simulink library "DC_Loads_Lib"  (R2021b)
settings: Solver=VariableStepAuto  StartTime=0.0  StopTime=10.0  RelTol=1e-3
undefined symbols (not defined in the file): APN_Param, D1, Delta, Hydride, Metal, Nickel, Ts
libraries: fl_lib x27, nesl_utility x14, spsSeriesRLCBranchLib x8, spsIdealSwitchLib x4, spsCurrentMeasurementLib x4, spsGroundLib x4, spsUniversalBridgeLib x4, spsThreePhaseTransformerThreeWindingsLib x2, spsBatteryLib x1, simulink x1, spsDCMachineLib x1, spsVoltageMeasurementLib x1
Description:
  | Copyright 2019-2021 The MathWorks, Inc.
settings Model: Creator=smiller  LastModifiedBy=janvan
settings SolverCC: AlgebraicLoopSolver=TrustRegion
settings DebuggingCC: SFMachineParentedDataDiag=warning
settings SFSimCC: CustomCodeUndefinedFunction=UseInterfaceOnly

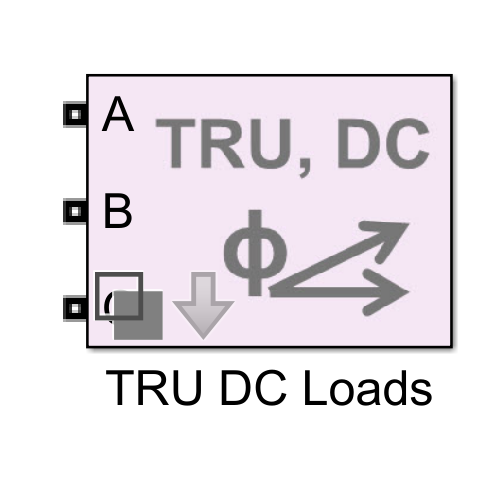
[thumbnail: Simulink's stored preview of the top-level diagram]
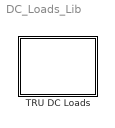
== system DC_Loads_Lib ==
  TRU DC Loads : Subsystem  RequirementInfo={} %GIDa_9ca9392e_c8fd_4c90_afb4_e22deb55bae6  Variant=on  VariantControlMode=label  LabelModeActiveChoice=Phasor  mask{ModelType=Phasor, PQ_Model=Initial}
      mask prompts: ModelType "Model Type"; PQ_Model "PQ Model"
      mask init:
      | set_param(gcb,'LabelModeActiveChoice',get_param(gcb,'ModelType'));
      | set_param([gcb '/Phasor'],'PQ_Model',get_param(gcb,'PQ_Model'));
      settings: AttributesFormatString=%<BlockChoice>
      mask TypeOptions ModelType: Detailed | Multidomain | Phasor
      mask TypeOptions PQ_Model: Initial | Tuned
      mask Display:
      | blk=find_system(gcbh, 'SearchDepth', 1, 'FollowLinks','on','LookUnderMasks','all', 'Parent', gcb,'VariantObject', get_param(gcb,'activevariant'));
      | eval(get_param(blk, 'MaskDisplay'));

== system DC_Loads_Lib/TRU DC Loads ==
  Detailed : Subsystem  VariantControl=Detailed
      mask Display: image('TRU_Detailed_IMAGE.jpg');
  Multidomain : Subsystem  VariantControl=Multidomain
      mask Display: image('TRU_Multidomain_IMAGE.jpg');
  Phasor : Subsystem  VariantControl=Phasor  mask{PQ_Model=Initial}
      mask prompts: PQ_Model "PQ Model"
      mask init:
      | set_param([gcb '/Calc PQ'],'PQ_Model',get_param(gcb,'PQ_Model'));
      mask TypeOptions PQ_Model: Initial | Tuned
      mask Display: image('TRU_Phasor_IMAGE.jpg');
  A : PMIOPort  Side=Left
  B : PMIOPort  Port=2  Side=Left
  C : PMIOPort  Port=3  Side=Left

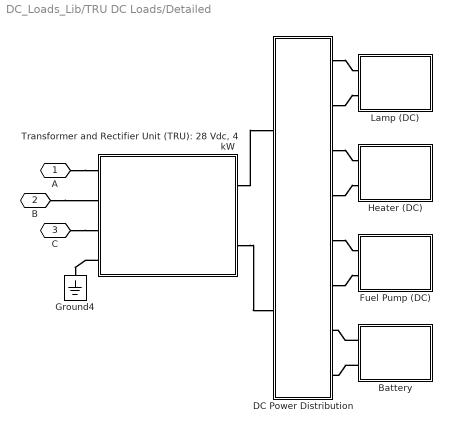
== system DC_Loads_Lib/TRU DC Loads/Detailed ==
  Battery : Subsystem
      mask Display:
      | image(imread('BatteryDC_PS_IMAGE.jpg','jpg'))
      | port_label('LConn',1,'+');
      | port_label('LConn',2,'-');
  "DC Power Distribution " : Subsystem
  Fuel Pump (DC) : Subsystem
      mask Display:
      | image(imread('PumpDC_PS_IMAGE.jpg','jpg'))
      | port_label('LConn',1,'+');
      | port_label('LConn',2,'-');
  Ground4 : spsGroundLib/Ground  LConnTagsString=a
  Heater (DC) : Subsystem
      mask Display:
      | image(imread('HeaterDC_PS_IMAGE.jpg','jpg'))
      | port_label('LConn',1,'+');
      | port_label('LConn',2,'-');
  Lamp (DC) : Subsystem
      mask Display:
      | image(imread('LampDC_PS_IMAGE.jpg','jpg'))
      | port_label('LConn',1,'+');
      | port_label('LConn',2,'-');
  "Transformer and Rectifier Unit (TRU): 28 Vdc, 4 kW" : Subsystem
      mask Display:
      | image(imread('TRU_PS_IMAGE.jpg','jpg'));
      | port_label('LConn',1,'A');
      | port_label('LConn',2,'B');
      | port_label('LConn',3,'C');
      | port_label('LConn',4,'N');
      | port_label('RConn',1,'+');
      | port_label('RConn',2,'-');
  A : PMIOPort  Side=Left
  B : PMIOPort  Port=2  Side=Left
  C : PMIOPort  Port=3  Side=Left
  connections:
  A/RConn1 -- "Transformer and Rectifier Unit (TRU): 28 Vdc, 4 kW"/LConn1
  C/RConn1 -- "Transformer and Rectifier Unit (TRU): 28 Vdc, 4 kW"/LConn3
  B/RConn1 -- "Transformer and Rectifier Unit (TRU): 28 Vdc, 4 kW"/LConn2
  "Transformer and Rectifier Unit (TRU): 28 Vdc, 4 kW"/RConn2 -- "DC Power Distribution "/LConn2
  "DC Power Distribution "/RConn6 -- Fuel Pump (DC)/LConn2
  "DC Power Distribution "/RConn1 -- Lamp (DC)/LConn1
  "DC Power Distribution "/RConn5 -- Fuel Pump (DC)/LConn1
  "DC Power Distribution "/RConn2 -- Lamp (DC)/LConn2
  "Transformer and Rectifier Unit (TRU): 28 Vdc, 4 kW"/RConn1 -- "DC Power Distribution "/LConn1
  "Transformer and Rectifier Unit (TRU): 28 Vdc, 4 kW"/LConn4 -- Ground4/LConn1
  "DC Power Distribution "/RConn3 -- Heater (DC)/LConn1
  "DC Power Distribution "/RConn4 -- Heater (DC)/LConn2
  Battery/LConn1 -- "DC Power Distribution "/RConn7
  Battery/LConn2 -- "DC Power Distribution "/RConn8

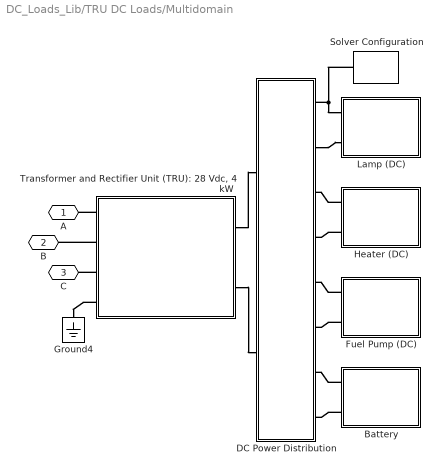
== system DC_Loads_Lib/TRU DC Loads/Multidomain ==
  Battery : Subsystem
      mask Display:
      | image(imread('BatteryDC_SS_IMAGE.jpg','jpg'))
      | port_label('LConn',1,'+');
      | port_label('LConn',2,'-');
  "DC Power Distribution " : Subsystem
  Fuel Pump (DC) : Subsystem
      mask Display:
      | image(imread('PumpDC_SS_IMAGE.jpg','jpg'))
      | port_label('LConn',1,'+');
      | port_label('LConn',2,'-');
  Ground4 : spsGroundLib/Ground  LConnTagsString=a
  Heater (DC) : Subsystem
      mask Display:
      | image(imread('HeaterDC_SS_IMAGE.jpg','jpg'))
      | port_label('LConn',1,'+');
      | port_label('LConn',2,'-');
  Lamp (DC) : Subsystem
      mask Display:
      | image(imread('LampDC_SS_IMAGE.jpg','jpg'))
      | port_label('LConn',1,'+');
      | port_label('LConn',2,'-');
  Solver Configuration : nesl_utility/Solver Configuration  PhysicalDomain=network_engine_domain  SubClassName=solver  LeftPortType=input  RightPortType=generic  Tones=[]  Harmonics=[]  SimulateNoise=off  Profile=off  UseLocalSampling=off  EnableSwitchedLinearOptims=on  FrequencyDomain=off  UseCCode=off  RelTol=0.001  AbsTol=1e-06  MinStep=1e-09  ToWorkspace=off  RevertToSquareIcSolve=off  NumHomotopyIterations=100  PhasorMode=off  PhasorModeNumHarmonics=1  DoDC=off  ResidualTolerance=1e-9  UseLocalSolver=on  LocalSolverChoice=NE_BACKWARD_EULER_ADVANCER  LocalSolverSampleTime=Ts  DoFixedCost=on  MaxNonlinIter=3  MaxModeIter=2  ComputeImpulses=off  ImpulseIterations=2  LinearAlgebra=Sparse  EquationFormulation=NE_TIME_EF  DelaysMemoryBudget=1024  AutomaticFiltering=on  FilteringTimeConstant=0.001  PartitionStorageMethod=AS_NEEDED  PartitionMemoryBudget=1024  PartitionMethod=FAST
      settings: SourceProductBaseCode=PW,SS
  "Transformer and Rectifier Unit (TRU): 28 Vdc, 4 kW" : Subsystem
      mask Display:
      | image(imread('TRU_PSSS_IMAGE.jpg','jpg'));
      | port_label('LConn',1,'A');
      | port_label('LConn',2,'B');
      | port_label('LConn',3,'C');
      | port_label('LConn',4,'N');
      | port_label('RConn',1,'+');
      | port_label('RConn',2,'-');
  A : PMIOPort  Side=Left
  B : PMIOPort  Port=2  Side=Left
  C : PMIOPort  Port=3  Side=Left
  connections:
  Battery/LConn2 -- "DC Power Distribution "/RConn8
  Battery/LConn1 -- "DC Power Distribution "/RConn7
  "Transformer and Rectifier Unit (TRU): 28 Vdc, 4 kW"/RConn2 -- "DC Power Distribution "/LConn2
  "Transformer and Rectifier Unit (TRU): 28 Vdc, 4 kW"/RConn1 -- "DC Power Distribution "/LConn1
  Fuel Pump (DC)/LConn1 -- "DC Power Distribution "/RConn5
  Fuel Pump (DC)/LConn2 -- "DC Power Distribution "/RConn6
  Heater (DC)/LConn1 -- "DC Power Distribution "/RConn3
  Heater (DC)/LConn2 -- "DC Power Distribution "/RConn4
  "DC Power Distribution "/RConn1 -- Lamp (DC)/LConn1 -- Solver Configuration/RConn1
  "DC Power Distribution "/RConn2 -- Lamp (DC)/LConn2
  "Transformer and Rectifier Unit (TRU): 28 Vdc, 4 kW"/LConn1 -- A/RConn1
  "Transformer and Rectifier Unit (TRU): 28 Vdc, 4 kW"/LConn3 -- C/RConn1
  "Transformer and Rectifier Unit (TRU): 28 Vdc, 4 kW"/LConn2 -- B/RConn1
  "Transformer and Rectifier Unit (TRU): 28 Vdc, 4 kW"/LConn4 -- Ground4/LConn1

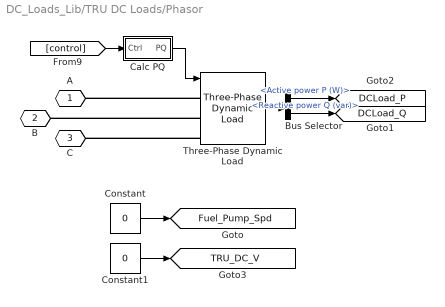
== system DC_Loads_Lib/TRU DC Loads/Phasor ==
  Bus Selector : BusSelector  OutputSignals=Active power P (W),Reactive power Q (var)
  Calc PQ : Subsystem  Variant=on  VariantControlMode=label  LabelModeActiveChoice=Initial  mask{PQ_Model=Initial}
      mask prompts: PQ_Model "PQ Model"
      mask init:
      | set_param(gcb,'LabelModeActiveChoice',get_param(gcb,'PQ_Model'));
      settings: AttributesFormatString=%<LabelModeActiveChoice>
      mask TypeOptions PQ_Model: Initial | Tuned
  Constant : Constant  Value=0
  Constant1 : Constant  Value=0
  Three-Phase Dynamic Load : spsThreePhaseDynamicLoadLib/Three-Phase Dynamic Load  NominalVoltage=[ 500e3 400 ]  ActiveReactivePowers=[APN_Param.TRU.P APN_Param.TRU.Q]  PositiveSequence=[0.0004 0]  ExternalControl=on  NpNq=[1.3 2]  TimeConstants="[0  0  0  0]"  MinimumVoltage=0.7  Tfilter=1e-4  LoadFlowParameters=[4 0 0 0 0]
      settings: SourceProductBaseCode=PS
  A : PMIOPort  Side=Left
  B : PMIOPort  Port=2  Side=Left
  C : PMIOPort  Port=3  Side=Left
  tag scope: DCLoad_P=global, DCLoad_Q=global, Fuel_Pump_Spd=global, TRU_DC_V=global
  wires:
  Bus Selector/1 -> [DCLoad_P]  "<Active power P (W)>"
  Three-Phase Dynamic Load/1 -> Bus Selector/1
  Constant/1 -> [Fuel_Pump_Spd]
  Bus Selector/2 -> [DCLoad_Q]  "<Reactive power Q (var)>"
  [control] -> Calc PQ/1(Ctrl)
  Calc PQ/1(PQ) -> Three-Phase Dynamic Load/1
  Constant1/1 -> [TRU_DC_V]
  connections:
  Three-Phase Dynamic Load/LConn3 -- C/RConn1
  Three-Phase Dynamic Load/LConn2 -- B/RConn1
  Three-Phase Dynamic Load/LConn1 -- A/RConn1

== system DC_Loads_Lib/TRU DC Loads/Detailed/Battery ==
  Battery : spsBatteryLib/Battery  BatType=Nickel-Metal-Hydride  ShowTempParam=off  ThermalPreset=no  ShowAgeParam=off  NomV=28  NomQ=12  SOC=100  Batt_Tr=30  PresetModel=on  MaxQ=12.9231  MinV=21  FullV=32.9831  Dis_rate=2.4  R=0.023333  Normal_OP=11.5385  expZone="[30.3729          2.4]"  current=[1.5 3]  Units=Ampere-hour  Tci=20  NomT=20  T2=-30  MaxQ2=4.8  FullV2=7.1  Normal_OP2=5.72  expZone2="[6.58  1]"  Rca=0.6  ti=1000  Dp=0  Neq0=0  Tsim=1e6  Ta1=25  Qeol=5.4*0.9  Reol=0.013333*1.2  Char_age=[2.3478, 3]  Dis_age=[2.3478, 10]  N1=1500  N2=10500  N3=1000  N4=1400  Ta2=45  N5=950
  Terminator : Terminator
  + : PMIOPort  Side=Left
  - : PMIOPort  Port=2  Side=Left
  wires:
  Battery/1 -> Terminator/1
  connections:
  Battery/LConn1 -- +/RConn1
  Battery/LConn2 -- -/RConn1

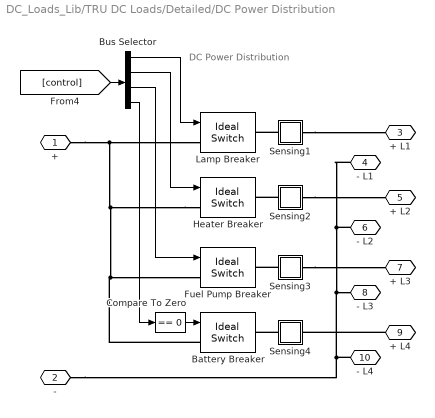
== system DC_Loads_Lib/TRU DC Loads/Detailed/DC Power Distribution  ==
  note: DC Power Distribution
  Battery Breaker : spsIdealSwitchLib/Ideal Switch  Ron=0.001  Lon=0  IC=0  Rs=1e3  Cs=inf  Measurements=off
  Bus Selector : BusSelector  OutputSignals=TRU_B_Bus.DC_Lamp_B,TRU_B_Bus.DC_Heater_B,TRU_B_Bus.DC_Pump_B,TRU_B
  Compare To Zero : simulink/Logic and Bit Operations/Compare To Zero  relop===  OutDataTypeStr=boolean
  Fuel Pump Breaker : spsIdealSwitchLib/Ideal Switch  Ron=0.001  Lon=0  IC=0  Rs=1e3  Cs=inf  Measurements=off
  Heater Breaker : spsIdealSwitchLib/Ideal Switch  Ron=0.001  Lon=0  IC=0  Rs=1e3  Cs=inf  Measurements=off
  Lamp Breaker : spsIdealSwitchLib/Ideal Switch  Ron=0.001  Lon=0  IC=0  Rs=1e3  Cs=inf  Measurements=off
  Sensing1 : Subsystem
      mask Display: disp('S');
  Sensing2 : Subsystem
      mask Display: disp('S');
  Sensing3 : Subsystem
      mask Display: disp('S');
  Sensing4 : Subsystem
      mask Display: disp('S');
  + : PMIOPort  Side=Left
  - : PMIOPort  Port=2  Side=Left
  + L1 : PMIOPort  Port=3  Side=Right
  - L1 : PMIOPort  Port=4  Side=Right
  + L2 : PMIOPort  Port=5  Side=Right
  - L2 : PMIOPort  Port=6  Side=Right
  + L3 : PMIOPort  Port=7  Side=Right
  - L3 : PMIOPort  Port=8  Side=Right
  + L4 : PMIOPort  Port=9  Side=Right
  - L4 : PMIOPort  Port=10  Side=Right
  wires:
  Bus Selector/3 -> Fuel Pump Breaker/1
  Bus Selector/2 -> Heater Breaker/1
  Bus Selector/1 -> Lamp Breaker/1
  [control] -> Bus Selector/1
  Bus Selector/4 -> Compare To Zero/1
  Compare To Zero/1 -> Battery Breaker/1
  connections:
  - L2/RConn1 -- - L1/RConn1 -- - L3/RConn1 -- - L4/RConn1 -- -/RConn1
  Heater Breaker/LConn1 -- Battery Breaker/LConn1 -- Fuel Pump Breaker/LConn1 -- Lamp Breaker/LConn1 -- +/RConn1
  Sensing1/LConn1 -- Lamp Breaker/RConn1
  Sensing1/RConn1 -- + L1/RConn1
  Sensing2/LConn1 -- Heater Breaker/RConn1
  Sensing2/RConn1 -- + L2/RConn1
  Sensing3/LConn1 -- Fuel Pump Breaker/RConn1
  Sensing3/RConn1 -- + L3/RConn1
  Sensing4/LConn1 -- Battery Breaker/RConn1
  + L4/RConn1 -- Sensing4/RConn1

== system DC_Loads_Lib/TRU DC Loads/Detailed/Fuel Pump (DC) ==
  Bus Selector : BusSelector  OutputSignals=Speed wm (rad/s)
  DC Machine : spsDCMachineLib/DC Machine  PresetModel=No  MechanicalLoad=Torque TL  FieldType=Wound  ShowDetailedParameters=on  MeasurementBus=off  RLa=[ .35 0.0001]  RLf="[ 240  12]"  Laf=1  MachineConstant=Torque constant (N.m/A)  Ke=1.8  Kt=1.8  J=0.0005  Bm=0  Tf=0  w0=0  Ifinit=0  TsPowergui=0  TsBlock=-1
  Gain : Gain  Gain=1.5/200
  + : PMIOPort  Side=Left
  - : PMIOPort  Port=2  Side=Left
  tag scope: Fuel_Pump_Spd=global
  wires:
  Bus Selector/1 -> Gain/1, [Fuel_Pump_Spd]  "<Speed wm (rad/s)>"
  DC Machine/1 -> Bus Selector/1
  Gain/1 -> DC Machine/1
  connections:
  DC Machine/LConn2 -- DC Machine/LConn1 -- +/RConn1
  DC Machine/RConn2 -- DC Machine/RConn1 -- -/RConn1

== system DC_Loads_Lib/TRU DC Loads/Detailed/Heater (DC) ==
  note: DC Load
  Series RLC Branch3 : spsSeriesRLCBranchLib/Series RLC Branch  LConnTagsString=__new0  RConnTagsString=__new0  BranchType=R  Resistance=1  Inductance=[]  SetiL0=off  InitialCurrent=0  Capacitance=[]  Setx0=off  InitialVoltage=0  Measurements=Branch voltage and current
  + : PMIOPort  Side=Left
  - : PMIOPort  Port=2  Side=Left
  connections:
  +/RConn1 -- Series RLC Branch3/LConn1
  -/RConn1 -- Series RLC Branch3/RConn1

== system DC_Loads_Lib/TRU DC Loads/Detailed/Lamp (DC) ==
  note: DC Load
  Series RLC Branch3 : spsSeriesRLCBranchLib/Series RLC Branch  LConnTagsString=__new0  RConnTagsString=__new0  BranchType=R  Resistance=1  Inductance=[]  SetiL0=off  InitialCurrent=0  Capacitance=[]  Setx0=off  InitialVoltage=0  Measurements=Branch voltage and current
  + : PMIOPort  Side=Left
  - : PMIOPort  Port=2  Side=Left
  connections:
  -/RConn1 -- Series RLC Branch3/RConn1
  +/RConn1 -- Series RLC Branch3/LConn1

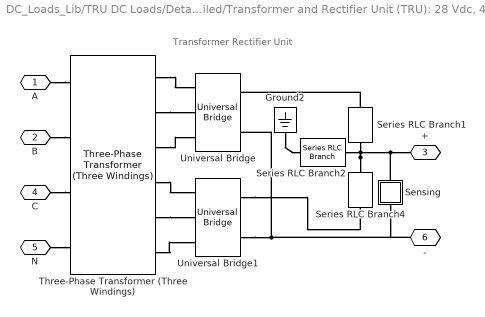
== system DC_Loads_Lib/TRU DC Loads/Detailed/Transformer and Rectifier Unit (TRU): 28 Vdc, 4 kW ==
  note: Transformer Rectifier Unit
  Ground2 : spsGroundLib/Ground  LConnTagsString=a
  Sensing : Subsystem
  Series RLC Branch1 : spsSeriesRLCBranchLib/Series RLC Branch  LConnTagsString=__new0  RConnTagsString=__new0  BranchType=L  Resistance=[]  Inductance=2e-3  SetiL0=on  InitialCurrent=0  Capacitance=[]  Setx0=off  InitialVoltage=0  Measurements=Branch voltage and current
  Series RLC Branch2 : spsSeriesRLCBranchLib/Series RLC Branch  LConnTagsString=__new0  RConnTagsString=__new0  BranchType=C  Resistance=[]  Inductance=[]  SetiL0=off  InitialCurrent=0  Capacitance=1e-6  Setx0=off  InitialVoltage=0  Measurements=None
  Series RLC Branch4 : spsSeriesRLCBranchLib/Series RLC Branch  LConnTagsString=__new0  RConnTagsString=__new0  BranchType=L  Resistance=[]  Inductance=2e-3  SetiL0=off  InitialCurrent=0  Capacitance=[]  Setx0=off  InitialVoltage=0  Measurements=Branch voltage and current
  Three-Phase Transformer (Three Windings) : spsThreePhaseTransformerThreeWindingsLib/Three-Phase Transformer (Three Windings)  Winding1Connection=Yn  Winding2Connection=Delta (D1)  Winding3Connection=Delta (D1)  CoreType=Three single-phase transformers  SetSaturation=off  Hysteresis=off  DataFile='hysteresis'  SetInitialFlux=off  Measurements=None  UNITS=pu  NominalPower=[ 4200 , 400 ]  Winding1=[ 200 , 0.0002 , 0 ]  Winding2=[ 22 , 0.0002 , 0 ]  Winding3=[ 22 , 0.0002 , 0]  Rm=500  Lm=500*10  L0=0.5  Saturation=[ 0,0 ; 0.0024,1.2 ; 1.0,1.52 ]  InitialFluxes=[0.8 -0.8 0.7]  BreakLoop=off  DiscreteSolver=Trapezoidal iterative  DataType=off  TransfoNumber=0
      settings: SourceProductBaseCode=PS
  Universal Bridge : spsUniversalBridgeLib/Universal Bridge  Arms=3  SnubberResistance=1e3  SnubberCapacitance=1e-6  Device=Diodes  Ron=1e-3  Lon=0  ForwardVoltages="[  0  0  ]"  ForwardVoltage=0.8  GTOparameters=[ 10e-6 , 20e-6 ]  IGBTparameters=[ 1e-6 , 2e-6 ]  Measurements=None  Measurements_2=None  converterType=Rectifier
  Universal Bridge1 : spsUniversalBridgeLib/Universal Bridge  Arms=3  SnubberResistance=1e3  SnubberCapacitance=1e-6  Device=Diodes  Ron=1e-3  Lon=0  ForwardVoltages="[  0  0  ]"  ForwardVoltage=0.8  GTOparameters=[ 10e-6 , 20e-6 ]  IGBTparameters=[ 1e-6 , 2e-6 ]  Measurements=None  Measurements_2=None  converterType=Rectifier
  A : PMIOPort  Side=Left
  B : PMIOPort  Port=2  Side=Left
  + : PMIOPort  Port=3  Side=Right
  C : PMIOPort  Port=4  Side=Left
  N : PMIOPort  Port=5  Side=Left
  - : PMIOPort  Port=6  Side=Right
  connections:
  Universal Bridge1/RConn1 -- Series RLC Branch4/RConn1
  Three-Phase Transformer (Three Windings)/RConn6 -- Universal Bridge1/LConn3
  Three-Phase Transformer (Three Windings)/RConn5 -- Universal Bridge1/LConn2
  Three-Phase Transformer (Three Windings)/RConn4 -- Universal Bridge1/LConn1
  Series RLC Branch4/LConn1 -- Sensing/RConn1 -- +/RConn1 -- Series RLC Branch2/LConn1 -- Series RLC Branch1/RConn1
  Series RLC Branch1/LConn1 -- Universal Bridge/RConn1
  N/RConn1 -- Three-Phase Transformer (Three Windings)/LConn4
  C/RConn1 -- Three-Phase Transformer (Three Windings)/LConn3
  B/RConn1 -- Three-Phase Transformer (Three Windings)/LConn2
  A/RConn1 -- Three-Phase Transformer (Three Windings)/LConn1
  Three-Phase Transformer (Three Windings)/RConn3 -- Universal Bridge/LConn3
  Three-Phase Transformer (Three Windings)/RConn2 -- Universal Bridge/LConn2
  Three-Phase Transformer (Three Windings)/RConn1 -- Universal Bridge/LConn1
  Universal Bridge1/RConn2 -- -/RConn1 -- Sensing/LConn1 -- Universal Bridge/RConn2
  Ground2/LConn1 -- Series RLC Branch2/RConn1

== system DC_Loads_Lib/TRU DC Loads/Multidomain/Battery ==
  Ambient temperature : fl_lib/Physical Signals/Sources/PS Constant  constant=273+25
  Battery cell : APN_Battery_Lib/Battery cell  SystemSampleTime=-1  VariantActivationTime=update diagram  Latency=0  AutoFrameSizeCalculation=off
  Convective Heat Transfer : fl_lib/Thermal/Thermal Elements/Convective Heat Transfer  area=Area m^2  heat_tr_coeff=Rtheta W/(m^2 * K)  T_specify=off  T_priority=High  T=0 K  T_nominal_specify=off  T_nominal_unit=K  T_nominal_value=1  Q_specify=off  Q_priority=High  Q=0 J/s  Q_nominal_specify=off  Q_nominal_unit=J/s  Q_nominal_value=1
  Ideal Temperature Source : fl_lib/Thermal/Thermal Sources/Controlled Temperature Source
  Thermal Reference : fl_lib/Thermal/Thermal Elements/Thermal Reference
  + : PMIOPort  Side=Left
  - : PMIOPort  Port=2  Side=Left
  connections:
  Battery cell/RConn1 -- -/RConn1
  +/RConn1 -- Battery cell/LConn1
  Thermal Reference/LConn1 -- Ideal Temperature Source/RConn2
  Ideal Temperature Source/RConn1 -- Ambient temperature/RConn1
  Ideal Temperature Source/LConn1 -- Convective Heat Transfer/LConn1
  Convective Heat Transfer/RConn1 -- Battery cell/LConn2

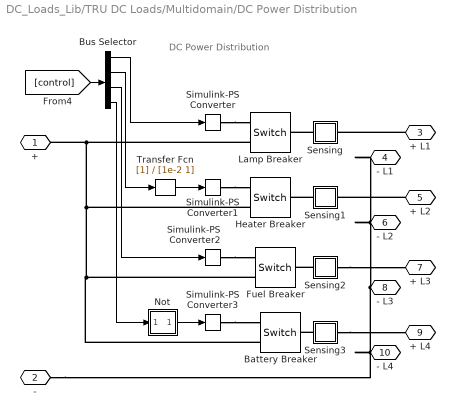
== system DC_Loads_Lib/TRU DC Loads/Multidomain/DC Power Distribution  ==
  note: DC Power Distribution
  Battery Breaker : fl_lib/Electrical/Electrical Elements/Switch  R_closed=0.001 Ohm  G_open=1e-8 1/Ohm  Threshold=0  i_specify=off  i_priority=High  i=0 A  i_nominal_specify=off  i_nominal_unit=A  i_nominal_value=1  v_specify=off  v_priority=High  v=0 V  v_nominal_specify=off  v_nominal_unit=V  v_nominal_value=1
  Bus Selector : BusSelector  OutputSignals=TRU_B_Bus.DC_Lamp_B,TRU_B_Bus.DC_Heater_B,TRU_B_Bus.DC_Pump_B,TRU_B
  Fuel Breaker : fl_lib/Electrical/Electrical Elements/Switch  R_closed=0.001 Ohm  G_open=1e-8 1/Ohm  Threshold=0  i_specify=off  i_priority=High  i=0 A  i_nominal_specify=off  i_nominal_unit=A  i_nominal_value=1  v_specify=off  v_priority=High  v=0 V  v_nominal_specify=off  v_nominal_unit=V  v_nominal_value=1
  Heater Breaker : fl_lib/Electrical/Electrical Elements/Switch  R_closed=0.001 Ohm  G_open=1e-8 1/Ohm  Threshold=0  i_specify=off  i_priority=High  i=0 A  i_nominal_specify=off  i_nominal_unit=A  i_nominal_value=1  v_specify=off  v_priority=High  v=0 V  v_nominal_specify=off  v_nominal_unit=V  v_nominal_value=1
  Lamp Breaker : fl_lib/Electrical/Electrical Elements/Switch  R_closed=0.001 Ohm  G_open=1e-8 1/Ohm  Threshold=0  i_specify=off  i_priority=High  i=0 A  i_nominal_specify=off  i_nominal_unit=A  i_nominal_value=1  v_specify=off  v_priority=High  v=0 V  v_nominal_specify=off  v_nominal_unit=V  v_nominal_value=1
  Not : Subsystem
      mask Display: disp('Not')
  Sensing : Subsystem
      mask Display: disp('S');
  Sensing1 : Subsystem
      mask Display: disp('S');
  Sensing2 : Subsystem
      mask Display: disp('S');
  Sensing3 : Subsystem
      mask Display: disp('S');
  Simulink-PS Converter{,1..3} (4 alike) : nesl_utility/Simulink-PS Converter  PhysicalDomain=network_engine_domain  SubClassName=ps_input  LeftPortType=input  RightPortType=output  PseudoPeriodic=off  Frequencies=[]  NoiseDistribution=none  NoiseParameters=[]  Unit=1  AffineConversion=off  FilteringAndDerivatives=zero  SimscapeFilterOrder=1  InputFilterTimeConstant=0.005  UdotUserProvided=1
      settings: SourceProductBaseCode=PW,SS
  Transfer Fcn : TransferFcn  Denominator=[1e-2 1]
  + : PMIOPort  Side=Left
  - : PMIOPort  Port=2  Side=Left
  + L1 : PMIOPort  Port=3  Side=Right
  - L1 : PMIOPort  Port=4  Side=Right
  + L2 : PMIOPort  Port=5  Side=Right
  - L2 : PMIOPort  Port=6  Side=Right
  + L3 : PMIOPort  Port=7  Side=Right
  - L3 : PMIOPort  Port=8  Side=Right
  + L4 : PMIOPort  Port=9  Side=Right
  - L4 : PMIOPort  Port=10  Side=Right
  wires:
  Transfer Fcn/1 -> Simulink-PS Converter1/1
  Not/1(Out1) -> Simulink-PS Converter3/1
  Bus Selector/4 -> Not/1(In1)
  [control] -> Bus Selector/1
  Bus Selector/1 -> Simulink-PS Converter/1
  Bus Selector/2 -> Transfer Fcn/1
  Bus Selector/3 -> Simulink-PS Converter2/1
  connections:
  Sensing3/LConn1 -- Battery Breaker/LConn1
  Sensing2/LConn1 -- Fuel Breaker/LConn1
  Simulink-PS Converter3/RConn1 -- Battery Breaker/RConn1
  Simulink-PS Converter2/RConn1 -- Fuel Breaker/RConn1
  Sensing1/LConn1 -- Heater Breaker/LConn1
  Simulink-PS Converter1/RConn1 -- Heater Breaker/RConn1
  + L1/RConn1 -- Sensing/RConn1
  +/RConn1 -- Heater Breaker/RConn2 -- Fuel Breaker/RConn2 -- Battery Breaker/RConn2 -- Lamp Breaker/RConn2
  Sensing/LConn1 -- Lamp Breaker/LConn1
  Simulink-PS Converter/RConn1 -- Lamp Breaker/RConn1
  Sensing3/RConn1 -- + L4/RConn1
  -/RConn1 -- - L4/RConn1 -- - L3/RConn1 -- - L1/RConn1 -- - L2/RConn1
  + L2/RConn1 -- Sensing1/RConn1
  Sensing2/RConn1 -- + L3/RConn1

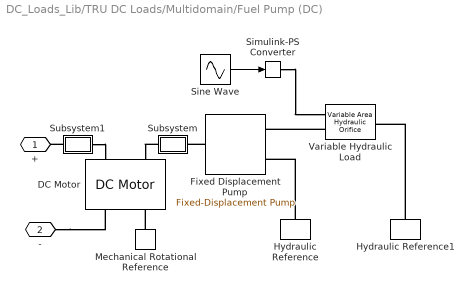
== system DC_Loads_Lib/TRU DC Loads/Multidomain/Fuel Pump (DC) ==
  DC Motor : ee_lib/Electromechanical/Brushed Motors/DC Motor  field_option=ee.enum.field_option.pm  Rf=100 Ohm  Lf=1 H  Laf=0.15 H  If0=0 A  parameterization=1  Ra=0.35 Ohm  La=1e-4 H  emf_or_torque=1  Kv=7.2e-5 V/rpm  Ki=6.876e-4 N*m/A  T_stall=2.4e-4 N*m  w_max=1.91e+4 rpm  w_rated=1.5e+4 rpm  P_rated=0.08 W  V_rated=1.5 V  lam_param=1  i_noload=0 A  V_i_noload=1.5 V  J=5e-4 kg*m^2  lam=1.5/200 N*m/(rad/s)  speed0=0 rpm  enable_fault_armature=simscape.enum.onoff.off  rev_faulted=1 / 3  G_faulted_armature=1e-5 S  fault_trigger_armature=ee.enum.faults.faultTrigger.temporal  t_fault_armature=1 s  max_permissible_current_armature=inf A  t_fail_on_current_armature=1 s  enable_fault_field=simscape.enum.onoff.off  G_faulted_field=1e-5 S  fault_trigger_field=ee.enum.faults.faultTrigger.temporal  t_fault_field=1 s  max_permissible_current_field=inf A  t_fail_on_current_field=1 s  fault_action=simscape.enum.assert.action.none  alpha=3.93e-3 1/K  Tmeas=25 degC  thermal_mass=100 J/K  initial_temperature=25 degC
  Fixed Displacement Pump : sh_lib/Pumps and Motors/Fixed-Displacement Pump  D=5e-6 m^3/rad  loss_spec=1  w_nominal=188 rad/s  pr_nominal=1e+7 Pa  visc_nominal=18 cSt  dens_nominal=900 kg/m^3  efficiency_vol=0.92  no_load_torque=0 N*m  torque_pressure_coeff=1*(5e-6)*((0.92)/(0.8)-1 ) N*m/Pa  p_diff_eff_TLU=[100000.0, 1000000.0, 2000000.0] Pa  omega_eff_TLU=[25.0, 50.0, 100.0, 200.0, 300.0, 400.0] rad/s  vol_eff_TLU=[0.816, 0.908, 0.954, 0.977, 0.981, 0.984; 0.325, 0.663, 0.831, 0.916, 0.925, 0.946; 0.137, 0.568, 0.78, 0.892, 0.893, 0.91]  mech_eff_TLU=[0.996, 0.996, 0.996, 0.996, 0.996, 0.996; 0.988, 0.989, 0.989, 0.989, 0.989, 0.99; 0.981, 0.981, 0.982, 0.982, 0.983, 0.984]  p_diff_loss_TLU=[100000.0, 1000000.0, 2000000.0] Pa  omega_loss_TLU=[25.0, 50.0, 100.0, 200.0, 300.0, 400.0] rad/s  vol_loss_TLU=[0.023, 0.023, 0.023, 0.023, 0.0285, 0.032; 0.0844, 0.0842, 0.0845, 0.084, 0.1125, 0.108; 0.1079, 0.108, 0.11, 0.108, 0.1605, 0.18] * 1e-3 m^3/s  mech_loss_TLU=[0.002, 0.002, 0.002, 0.002, 0.002, 0.002; 0.0607, 0.0556, 0.0556, 0.0556, 0.0556, 0.0505; 0.1937, 0.1937, 0.1833, 0.1833, 0.1729, 0.1626] N*m  pressure_threshold=1e5 Pa  omega_threshold=10 rad/s  quadrant_check=0  pressure_check=0  min_valid_pressure=0 Pa  vol_eff_min=1e-3  vol_eff_max=1  mech_eff_min=1e-3  mech_eff_max=1
      settings: SourceProductBaseCode=SH  InternalSimscapePortConfiguration="{\"Bottom\":[],\"Left\":[{\"id\":\"S\",\"label\":\"S\",\"type\":\"foundation.mechanical.rotational.rotational\"}],\"Right\":[{\"id\":\"P\",\"label\":\"P\",\"type\":\"foundation.hydraulic.hydraulic\"},{\"id\":\"T\",\"label\":\"T\",\"type\":\"foundation.hydraulic.hydraulic\"}],\"Top\":[]}"
  Hydraulic Reference : fl_lib/Hydraulic/Hydraulic Elements/Hydraulic Reference
  Hydraulic Reference1 : fl_lib/Hydraulic/Hydraulic Elements/Hydraulic Reference
  Mechanical Rotational Reference : fl_lib/Mechanical/Rotational Elements/Mechanical Rotational Reference
  Simulink-PS Converter : nesl_utility/Simulink-PS Converter  PhysicalDomain=network_engine_domain  SubClassName=ps_input  LeftPortType=input  RightPortType=output  PseudoPeriodic=off  Frequencies=[]  NoiseDistribution=none  NoiseParameters=[]  Unit=1  AffineConversion=off  FilteringAndDerivatives=filter  SimscapeFilterOrder=1  InputFilterTimeConstant=0.005  UdotUserProvided=1
      settings: SourceProductBaseCode=PW,SS
  Sine Wave : Sin  Amplitude=1e-4  Bias=1e-3  Frequency=2  SampleTime=0
  Subsystem : Subsystem
      mask Display: disp('S')
  Subsystem1 : Subsystem
      mask Display: disp('S')
  Variable Hydraulic Load : fl_lib/Hydraulic/Hydraulic Elements/Variable Area Hydraulic Orifice  C_d=0.7  min_area=1e-12 m^2  lam_spec=2  B_lam=0.999  Re_cr=12  q_specify=off  q_priority=High  q=1 m^3/s  q_nominal_specify=off  q_nominal_unit=m^3/s  q_nominal_value=1  p_specify=off  p_priority=High  p=0 Pa  p_nominal_specify=off  p_nominal_unit=Pa  p_nominal_value=1
      settings: SourceProductBaseCode=SS  InternalSimscapePortConfiguration="{\"Bottom\":[],\"Left\":[{\"id\":\"AR\",\"label\":\"AR\",\"type\":\"input\"},{\"id\":\"A\",\"label\":\"A\",\"type\":\"foundation.hydraulic.hydraulic\"}],\"Right\":[{\"id\":\"B\",\"label\":\"B\",\"type\":\"foundation.hydraulic.hydraulic\"}],\"Top\":[]}"
  + : PMIOPort  Side=Left
  - : PMIOPort  Port=2  Side=Left
  wires:
  Sine Wave/1 -> Simulink-PS Converter/1
  connections:
  Simulink-PS Converter/RConn1 -- Variable Hydraulic Load/LConn1
  Hydraulic Reference1/LConn1 -- Variable Hydraulic Load/RConn1
  Variable Hydraulic Load/LConn2 -- Fixed Displacement Pump/RConn1
  Hydraulic Reference/LConn1 -- Fixed Displacement Pump/RConn2
  Fixed Displacement Pump/LConn1 -- Subsystem/RConn1
  Subsystem1/RConn1 -- DC Motor/LConn1
  Subsystem1/LConn1 -- +/RConn1
  Subsystem/LConn1 -- DC Motor/LConn2
  Mechanical Rotational Reference/LConn1 -- DC Motor/RConn2
  -/RConn1 -- DC Motor/RConn1

== system DC_Loads_Lib/TRU DC Loads/Multidomain/Heater (DC) ==
  Atmosphere : fl_lib/Thermal/Thermal Elements/Thermal Reference
  Conductive Heat Transfer : fl_lib/Thermal/Thermal Elements/Conductive Heat Transfer  area=1e-4 m^2  thickness=0.1 m  th_cond=401 W/(m*K)  T_specify=off  T_priority=High  T=0 K  T_nominal_specify=off  T_nominal_unit=K  T_nominal_value=1  Q_specify=off  Q_priority=High  Q=0 J/s  Q_nominal_specify=off  Q_nominal_unit=J/s  Q_nominal_value=1
  Convective Heat Transfer : fl_lib/Thermal/Thermal Elements/Convective Heat Transfer  area=1e-4 m^2  heat_tr_coeff=20 W/(m^2 * K)  T_specify=off  T_priority=High  T=0 K  T_nominal_specify=off  T_nominal_unit=K  T_nominal_value=1  Q_specify=off  Q_priority=High  Q=0 J/s  Q_nominal_specify=off  Q_nominal_unit=J/s  Q_nominal_value=1
  Thermal Resistor : fl_lib/Electrical/Electrical Elements/Thermal Resistor  R0=1 Ohm  T0=25 degC  alpha=5e-5 1/K  tc=10 s  K_d=0.001 W/K  T_specify=on  T_priority=High  T=300 K  T_nominal_specify=off  T_nominal_unit=K  T_nominal_value=1
      settings: SourceProductBaseCode=SS  InternalSimscapePortConfiguration="{\"Bottom\":[],\"Left\":[{\"id\":\"H\",\"label\":\"H\",\"type\":\"foundation.thermal.thermal\"},{\"id\":\"p\",\"label\":\"+\",\"type\":\"foundation.electrical.electrical\"}],\"Right\":[{\"id\":\"n\",\"label\":\"-\",\"type\":\"foundation.electrical.electrical\"}],\"Top\":[]}"
  Thermal Mass : fl_lib/Thermal/Thermal Elements/Thermal Mass  mass=1 kg  sp_heat=447 J/kg/K  T_specify=on  T_priority=High  T=300 K  T_nominal_specify=off  T_nominal_unit=K  T_nominal_value=1  Q_specify=off  Q_priority=High  Q=0 J/s  Q_nominal_specify=off  Q_nominal_unit=J/s  Q_nominal_value=1
  + : PMIOPort  Side=Left
  - : PMIOPort  Port=2  Side=Left
  connections:
  Conductive Heat Transfer/LConn1 -- Thermal Resistor/LConn1
  Atmosphere/LConn1 -- Convective Heat Transfer/RConn1
  Conductive Heat Transfer/RConn1 -- Convective Heat Transfer/LConn1 -- Thermal Mass/LConn1
  +/RConn1 -- Thermal Resistor/LConn2
  -/RConn1 -- Thermal Resistor/RConn1

== system DC_Loads_Lib/TRU DC Loads/Multidomain/Lamp (DC) ==
  Simulink-PS Converter : nesl_utility/Simulink-PS Converter  PhysicalDomain=network_engine_domain  SubClassName=ps_input  LeftPortType=input  RightPortType=output  PseudoPeriodic=off  Frequencies=[]  NoiseDistribution=none  NoiseParameters=[]  Unit=1  AffineConversion=off  FilteringAndDerivatives=filter  SimscapeFilterOrder=1  InputFilterTimeConstant=0.005  UdotUserProvided=1
      settings: SourceProductBaseCode=PW,SS
  Sine Wave : Sin  Amplitude=0.25  Bias=1  Frequency=2  SampleTime=0
  Variable Resistor : fl_lib/Electrical/Electrical Elements/Variable Resistor  Rmin=0 Ohm  i_specify=off  i_priority=High  i=0 A  i_nominal_specify=off  i_nominal_unit=A  i_nominal_value=1  v_specify=off  v_priority=High  v=0 V  v_nominal_specify=off  v_nominal_unit=V  v_nominal_value=1
  + : PMIOPort  Side=Left
  - : PMIOPort  Port=2  Side=Left
  wires:
  Sine Wave/1 -> Simulink-PS Converter/1
  connections:
  Simulink-PS Converter/RConn1 -- Variable Resistor/LConn1
  -/RConn1 -- Variable Resistor/RConn1
  +/RConn1 -- Variable Resistor/LConn2

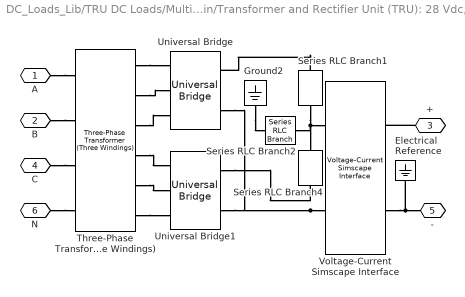
== system DC_Loads_Lib/TRU DC Loads/Multidomain/Transformer and Rectifier Unit (TRU): 28 Vdc, 4 kW ==
  Electrical Reference : fl_lib/Electrical/Electrical Elements/Electrical Reference
  Ground2 : spsGroundLib/Ground  LConnTagsString=a
  Series RLC Branch1 : spsSeriesRLCBranchLib/Series RLC Branch  LConnTagsString=__new0  RConnTagsString=__new0  BranchType=L  Resistance=[]  Inductance=2e-3  SetiL0=on  InitialCurrent=0  Capacitance=[]  Setx0=off  InitialVoltage=0  Measurements=Branch voltage and current
  Series RLC Branch2 : spsSeriesRLCBranchLib/Series RLC Branch  LConnTagsString=__new0  RConnTagsString=__new0  BranchType=C  Resistance=[]  Inductance=[]  SetiL0=off  InitialCurrent=0  Capacitance=1e-6  Setx0=off  InitialVoltage=0  Measurements=None
  Series RLC Branch4 : spsSeriesRLCBranchLib/Series RLC Branch  LConnTagsString=__new0  RConnTagsString=__new0  BranchType=L  Resistance=[]  Inductance=2e-3  SetiL0=off  InitialCurrent=0  Capacitance=[]  Setx0=off  InitialVoltage=0  Measurements=Branch voltage and current
  Three-Phase Transformer (Three Windings) : spsThreePhaseTransformerThreeWindingsLib/Three-Phase Transformer (Three Windings)  Winding1Connection=Yn  Winding2Connection=Delta (D1)  Winding3Connection=Delta (D1)  CoreType=Three single-phase transformers  SetSaturation=off  Hysteresis=off  DataFile='hysteresis'  SetInitialFlux=off  Measurements=None  UNITS=pu  NominalPower=[ 4200 , 400 ]  Winding1=[ 200 , 0.0002 , 0 ]  Winding2=[ 22 , 0.0002 , 0 ]  Winding3=[ 22 , 0.0002 , 0]  Rm=500  Lm=500*10  L0=0.5  Saturation=[ 0,0 ; 0.0024,1.2 ; 1.0,1.52 ]  InitialFluxes=[0.8 -0.8 0.7]  BreakLoop=off  DiscreteSolver=Trapezoidal iterative  DataType=off  TransfoNumber=0
      settings: SourceProductBaseCode=PS
  Universal Bridge : spsUniversalBridgeLib/Universal Bridge  Arms=3  SnubberResistance=1e3  SnubberCapacitance=1e-6  Device=Diodes  Ron=1e-3  Lon=0  ForwardVoltages="[  0  0  ]"  ForwardVoltage=0.8  GTOparameters=[ 10e-6 , 20e-6 ]  IGBTparameters=[ 1e-6 , 2e-6 ]  Measurements=None  Measurements_2=None  converterType=Rectifier
  Universal Bridge1 : spsUniversalBridgeLib/Universal Bridge  Arms=3  SnubberResistance=1e3  SnubberCapacitance=1e-6  Device=Diodes  Ron=1e-3  Lon=0  ForwardVoltages="[  0  0  ]"  ForwardVoltage=0.8  GTOparameters=[ 10e-6 , 20e-6 ]  IGBTparameters=[ 1e-6 , 2e-6 ]  Measurements=None  Measurements_2=None  converterType=Rectifier
  Voltage-Current Simscape Interface : spsVoltageCurrentSimscapeInterfaceLib/Voltage-Current Simscape Interface  DFT=off  Fmode=Unit delay (discrete)  T=1e-6  Ts=Ts  i0=0  v0=0  Sd=Specialized Power Systems side  Measurements=off
      settings: SourceProductBaseCode=PS
  A : PMIOPort  Side=Left
  B : PMIOPort  Port=2  Side=Left
  + : PMIOPort  Port=3  Side=Right
  C : PMIOPort  Port=4  Side=Left
  - : PMIOPort  Port=5  Side=Right
  N : PMIOPort  Port=6  Side=Left
  connections:
  Ground2/LConn1 -- Series RLC Branch2/RConn1
  Voltage-Current Simscape Interface/LConn2 -- Universal Bridge/RConn2 -- Universal Bridge1/RConn2
  Three-Phase Transformer (Three Windings)/RConn1 -- Universal Bridge/LConn1
  Three-Phase Transformer (Three Windings)/RConn2 -- Universal Bridge/LConn2
  Three-Phase Transformer (Three Windings)/RConn3 -- Universal Bridge/LConn3
  A/RConn1 -- Three-Phase Transformer (Three Windings)/LConn1
  B/RConn1 -- Three-Phase Transformer (Three Windings)/LConn2
  C/RConn1 -- Three-Phase Transformer (Three Windings)/LConn3
  Series RLC Branch1/LConn1 -- Universal Bridge/RConn1
  Voltage-Current Simscape Interface/LConn1 -- Series RLC Branch2/LConn1 -- Series RLC Branch4/LConn1 -- Series RLC Branch1/RConn1
  Three-Phase Transformer (Three Windings)/RConn4 -- Universal Bridge1/LConn1
  Three-Phase Transformer (Three Windings)/RConn5 -- Universal Bridge1/LConn2
  Three-Phase Transformer (Three Windings)/RConn6 -- Universal Bridge1/LConn3
  Universal Bridge1/RConn1 -- Series RLC Branch4/RConn1
  +/RConn1 -- Voltage-Current Simscape Interface/RConn1
  -/RConn1 -- Electrical Reference/LConn1 -- Voltage-Current Simscape Interface/RConn2
  N/RConn1 -- Three-Phase Transformer (Three Windings)/LConn4

== system DC_Loads_Lib/TRU DC Loads/Phasor/Calc PQ ==
  Ctrl : Inport
  Initial : Subsystem  VariantControl=Initial
  Tuned : Subsystem  VariantControl=Tuned
  PQ : Outport  VectorParamsAs1DForOutWhenUnconnected=off

== system DC_Loads_Lib/TRU DC Loads/Detailed/DC Power Distribution /Sensing1 ==
  Lamp Current Mmt. : spsCurrentMeasurementLib/Current Measurement  PhasorSimulation=off  OutputType=Complex  PSBequivalent=0
  + : PMIOPort  Side=Left
  - : PMIOPort  Port=2  Side=Right
  tag scope: DC_Lamp_I=global
  wires:
  Lamp Current Mmt./1 -> [DC_Lamp_I]
  connections:
  Lamp Current Mmt./RConn1 -- -/RConn1
  Lamp Current Mmt./LConn1 -- +/RConn1

== system DC_Loads_Lib/TRU DC Loads/Detailed/DC Power Distribution /Sensing2 ==
  Heater Current Mmt. : spsCurrentMeasurementLib/Current Measurement  PhasorSimulation=off  OutputType=Complex  PSBequivalent=0
  + : PMIOPort  Side=Left
  - : PMIOPort  Port=2  Side=Right
  tag scope: DC_Heater_I=global
  wires:
  Heater Current Mmt./1 -> [DC_Heater_I]
  connections:
  Heater Current Mmt./RConn1 -- -/RConn1
  Heater Current Mmt./LConn1 -- +/RConn1

== system DC_Loads_Lib/TRU DC Loads/Detailed/DC Power Distribution /Sensing3 ==
  Fuel Pump Current Mmt. : spsCurrentMeasurementLib/Current Measurement  PhasorSimulation=off  OutputType=Complex  PSBequivalent=0
  + : PMIOPort  Side=Left
  - : PMIOPort  Port=2  Side=Right
  tag scope: DC_Pump_I=global
  wires:
  Fuel Pump Current Mmt./1 -> [DC_Pump_I]
  connections:
  Fuel Pump Current Mmt./RConn1 -- -/RConn1
  Fuel Pump Current Mmt./LConn1 -- +/RConn1

== system DC_Loads_Lib/TRU DC Loads/Detailed/DC Power Distribution /Sensing4 ==
  Fuel Pump Current Mmt.1 : spsCurrentMeasurementLib/Current Measurement  PhasorSimulation=off  OutputType=Complex  PSBequivalent=0
  + : PMIOPort  Side=Left
  - : PMIOPort  Port=2  Side=Right
  tag scope: DC_Battery_I=global
  wires:
  Fuel Pump Current Mmt.1/1 -> [DC_Battery_I]
  connections:
  Fuel Pump Current Mmt.1/LConn1 -- +/RConn1
  -/RConn1 -- Fuel Pump Current Mmt.1/RConn1

== system DC_Loads_Lib/TRU DC Loads/Detailed/Transformer and Rectifier Unit (TRU): 28 Vdc, 4 kW/Sensing ==
  Voltage Measurement : spsVoltageMeasurementLib/Voltage Measurement  PhasorSimulation=off  OutputType=Complex  PSBequivalent=0
  + : PMIOPort  Side=Right
  - : PMIOPort  Port=2  Side=Left
  tag scope: TRU_DC_V=global
  wires:
  Voltage Measurement/1 -> [TRU_DC_V]
  connections:
  Voltage Measurement/LConn1 -- +/RConn1
  Voltage Measurement/LConn2 -- -/RConn1

== system DC_Loads_Lib/TRU DC Loads/Multidomain/DC Power Distribution /Not ==
  In1 : Inport
  Constant : Constant
  Gain : Gain  Gain=-1
  Sum : Sum  Inputs=|++
  Out1 : Outport  VectorParamsAs1DForOutWhenUnconnected=off
  wires:
  Constant/1 -> Sum/2
  Sum/1 -> Out1/1
  Gain/1 -> Sum/1
  In1/1 -> Gain/1

== system DC_Loads_Lib/TRU DC Loads/Multidomain/DC Power Distribution /Sensing ==
  Current Sensor : fl_lib/Electrical/Electrical Sensors/Current Sensor
  PS-Simulink Converter : nesl_utility/PS-Simulink Converter  PhysicalDomain=network_engine_domain  SubClassName=ps_output  LeftPortType=input  RightPortType=output  PseudoPeriodic=off  Frequencies=[]  Unit=1  AffineConversion=off
      settings: SourceProductBaseCode=PW,SS
  + : PMIOPort  Side=Left
  - : PMIOPort  Port=2  Side=Right
  tag scope: DC_Lamp_I=global
  wires:
  PS-Simulink Converter/1 -> [DC_Lamp_I]
  connections:
  Current Sensor/RConn2 -- -/RConn1
  Current Sensor/LConn1 -- +/RConn1
  PS-Simulink Converter/LConn1 -- Current Sensor/RConn1

== system DC_Loads_Lib/TRU DC Loads/Multidomain/DC Power Distribution /Sensing1 ==
  Current Sensor : fl_lib/Electrical/Electrical Sensors/Current Sensor
  PS-Simulink Converter : nesl_utility/PS-Simulink Converter  PhysicalDomain=network_engine_domain  SubClassName=ps_output  LeftPortType=input  RightPortType=output  PseudoPeriodic=off  Frequencies=[]  Unit=1  AffineConversion=off
      settings: SourceProductBaseCode=PW,SS
  + : PMIOPort  Side=Left
  - : PMIOPort  Port=2  Side=Right
  tag scope: DC_Heater_I=global
  wires:
  PS-Simulink Converter/1 -> [DC_Heater_I]
  connections:
  PS-Simulink Converter/LConn1 -- Current Sensor/RConn1
  Current Sensor/LConn1 -- +/RConn1
  Current Sensor/RConn2 -- -/RConn1

== system DC_Loads_Lib/TRU DC Loads/Multidomain/DC Power Distribution /Sensing2 ==
  Current Sensor : fl_lib/Electrical/Electrical Sensors/Current Sensor
  PS-Simulink Converter : nesl_utility/PS-Simulink Converter  PhysicalDomain=network_engine_domain  SubClassName=ps_output  LeftPortType=input  RightPortType=output  PseudoPeriodic=off  Frequencies=[]  Unit=1  AffineConversion=off
      settings: SourceProductBaseCode=PW,SS
  + : PMIOPort  Side=Left
  - : PMIOPort  Port=2  Side=Right
  tag scope: DC_Pump_I=global
  wires:
  PS-Simulink Converter/1 -> [DC_Pump_I]
  connections:
  Current Sensor/RConn2 -- -/RConn1
  Current Sensor/LConn1 -- +/RConn1
  PS-Simulink Converter/LConn1 -- Current Sensor/RConn1

== system DC_Loads_Lib/TRU DC Loads/Multidomain/DC Power Distribution /Sensing3 ==
  Current Sensor : fl_lib/Electrical/Electrical Sensors/Current Sensor
  PS-Simulink Converter : nesl_utility/PS-Simulink Converter  PhysicalDomain=network_engine_domain  SubClassName=ps_output  LeftPortType=input  RightPortType=output  PseudoPeriodic=off  Frequencies=[]  Unit=1  AffineConversion=off
      settings: SourceProductBaseCode=PW,SS
  + : PMIOPort  Side=Left
  - : PMIOPort  Port=2  Side=Right
  tag scope: DC_Battery_I=global
  wires:
  PS-Simulink Converter/1 -> [DC_Battery_I]
  connections:
  PS-Simulink Converter/LConn1 -- Current Sensor/RConn1
  Current Sensor/LConn1 -- +/RConn1
  Current Sensor/RConn2 -- -/RConn1

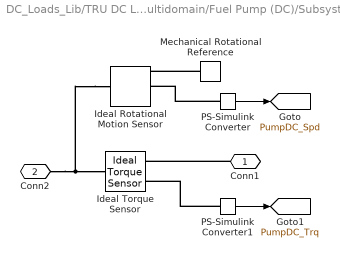
== system DC_Loads_Lib/TRU DC Loads/Multidomain/Fuel Pump (DC)/Subsystem ==
  Ideal Rotational Motion Sensor : fl_lib/Mechanical/Mechanical Sensors/Ideal Rotational Motion Sensor  wrap_angle=simscape.enum.onoff.off  offset=0 rad
  Ideal Torque Sensor : fl_lib/Mechanical/Mechanical Sensors/Ideal Torque Sensor
  Mechanical Rotational Reference : fl_lib/Mechanical/Rotational Elements/Mechanical Rotational Reference
  PS-Simulink Converter : nesl_utility/PS-Simulink Converter  PhysicalDomain=network_engine_domain  SubClassName=ps_output  LeftPortType=input  RightPortType=output  PseudoPeriodic=off  Frequencies=[]  Unit=1  AffineConversion=off
      settings: SourceProductBaseCode=PW,SS
  PS-Simulink Converter1 : nesl_utility/PS-Simulink Converter  PhysicalDomain=network_engine_domain  SubClassName=ps_output  LeftPortType=input  RightPortType=output  PseudoPeriodic=off  Frequencies=[]  Unit=1  AffineConversion=off
      settings: SourceProductBaseCode=PW,SS
  Conn1 : PMIOPort  Side=Right
  Conn2 : PMIOPort  Port=2  Side=Left
  tag scope: PumpDC_Spd=global, PumpDC_Trq=global
  wires:
  PS-Simulink Converter1/1 -> [PumpDC_Trq]
  PS-Simulink Converter/1 -> [PumpDC_Spd]
  connections:
  PS-Simulink Converter/LConn1 -- Ideal Rotational Motion Sensor/RConn2
  Mechanical Rotational Reference/LConn1 -- Ideal Rotational Motion Sensor/RConn1
  PS-Simulink Converter1/LConn1 -- Ideal Torque Sensor/RConn2
  Ideal Rotational Motion Sensor/LConn1 -- Ideal Torque Sensor/LConn1 -- Conn2/RConn1
  Conn1/RConn1 -- Ideal Torque Sensor/RConn1

== system DC_Loads_Lib/TRU DC Loads/Multidomain/Fuel Pump (DC)/Subsystem1 ==
  Current Sensor : fl_lib/Electrical/Electrical Sensors/Current Sensor
  PS-Simulink Converter1 : nesl_utility/PS-Simulink Converter  PhysicalDomain=network_engine_domain  SubClassName=ps_output  LeftPortType=input  RightPortType=output  PseudoPeriodic=off  Frequencies=[]  Unit=1  AffineConversion=off
      settings: SourceProductBaseCode=PW,SS
  Conn1 : PMIOPort  Side=Right
  Conn2 : PMIOPort  Port=2  Side=Left
  tag scope: PumpDC_i=global
  wires:
  PS-Simulink Converter1/1 -> [PumpDC_i]
  connections:
  Conn1/RConn1 -- Current Sensor/RConn2
  Conn2/RConn1 -- Current Sensor/LConn1
  PS-Simulink Converter1/LConn1 -- Current Sensor/RConn1

== system DC_Loads_Lib/TRU DC Loads/Phasor/Calc PQ/Initial ==
  Ctrl : Inport
  Bus Selector1 : BusSelector  OutputSignals=TRU_B
  Constant : Constant  Value=APN_Param.TRU.P
  Constant1 : Constant  Value=APN_Param.TRU.Q
  Filter : Subsystem  mask(First-order lag supporting vector signals){b=1e-2, x_initial=[APN_Param.TRU.P APN_Param.TRU.Q]*0}
      mask prompts: b "Filter time constant"; x_initial "Initial output"
      mask help: Models a lag of the form 1/(b*s+1) where s is the Laplace operator.
  Mux : Mux  Inputs=2
  Product : Product
  PQ : Outport  VectorParamsAs1DForOutWhenUnconnected=off
  wires:
  Constant1/1 -> Mux/2
  Constant/1 -> Mux/1
  Ctrl/1 -> Bus Selector1/1
  Mux/1 -> Product/1
  Bus Selector1/1 -> Product/2  "<TRU_B>"
  Filter/1(Out) -> PQ/1
  Product/1 -> Filter/1(In)

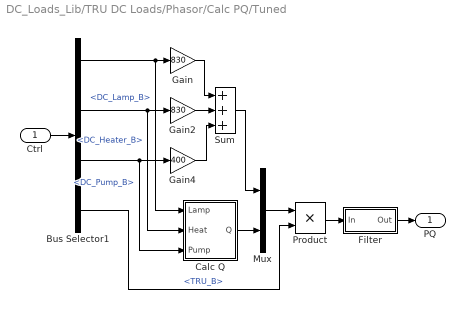
== system DC_Loads_Lib/TRU DC Loads/Phasor/Calc PQ/Tuned ==
  Ctrl : Inport
  Bus Selector1 : BusSelector  OutputSignals=TRU_B_Bus.DC_Lamp_B,TRU_B_Bus.DC_Heater_B,TRU_B_Bus.DC_Pump_B,TRU_B
  Calc Q : Subsystem
  Filter : Subsystem  mask(First-order lag supporting vector signals){b=1e-2, x_initial=0}
      mask prompts: b "Filter time constant"; x_initial "Initial output"
      mask help: Models a lag of the form 1/(b*s+1) where s is the Laplace operator.
  Gain : Gain  Gain=830
  Gain2 : Gain  Gain=830
  Gain4 : Gain  Gain=400
  Mux : Mux  Inputs=2
  Product : Product
  Sum : Sum  Inputs=+++
  PQ : Outport  VectorParamsAs1DForOutWhenUnconnected=off
  wires:
  Calc Q/1(Q) -> Mux/2
  Product/1 -> Filter/1(In)
  Filter/1(Out) -> PQ/1
  Bus Selector1/4 -> Product/2  "<TRU_B>"
  Gain4/1 -> Sum/3
  Gain2/1 -> Sum/2
  Gain/1 -> Sum/1
  Bus Selector1/3 -> Gain4/1, Calc Q/3(Pump)  "<DC_Pump_B>"
  Bus Selector1/2 -> Gain2/1, Calc Q/2(Heat)  "<DC_Heater_B>"
  Mux/1 -> Product/1
  Sum/1 -> Mux/1
  Bus Selector1/1 -> Gain/1, Calc Q/1(Lamp)  "<DC_Lamp_B>"
  Ctrl/1 -> Bus Selector1/1

== system DC_Loads_Lib/TRU DC Loads/Phasor/Calc PQ/Initial/Filter ==
  In : Inport
  Gain : Gain  Gain=1/b
  Integrator : Integrator  InitialCondition=x_initial
  Sum : Sum  Inputs=|+-  InputSameDT=on  SaturateOnIntegerOverflow=on  OutDataTypeStr=Inherit: Same as first input
  Out : Outport  VectorParamsAs1DForOutWhenUnconnected=off
  wires:
  Sum/1 -> Integrator/1
  In/1 -> Sum/1
  Integrator/1 -> Gain/1
  Gain/1 -> Sum/2, Out/1

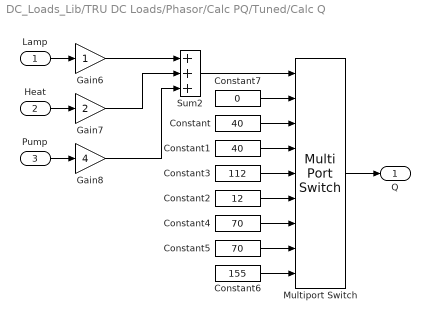
== system DC_Loads_Lib/TRU DC Loads/Phasor/Calc PQ/Tuned/Calc Q ==
  Lamp : Inport
  Heat : Inport  Port=2
  Pump : Inport  Port=3
  Constant : Constant  Value=40
  Constant1 : Constant  Value=40
  Constant2 : Constant  Value=12
  Constant3 : Constant  Value=112
  Constant4 : Constant  Value=70
  Constant5 : Constant  Value=70
  Constant6 : Constant  Value=155
  Constant7 : Constant  Value=0
  Gain6 : Gain
  Gain7 : Gain  Gain=2
  Gain8 : Gain  Gain=4
  Multiport Switch : MultiPortSwitch  DataPortOrder=Zero-based contiguous  Inputs=8  zeroidx=on
  Sum2 : Sum  Inputs=+++  OutDataTypeStr=int8
  Q : Outport  VectorParamsAs1DForOutWhenUnconnected=off
  wires:
  Heat/1 -> Gain7/1
  Lamp/1 -> Gain6/1
  Pump/1 -> Gain8/1
  Constant1/1 -> Multiport Switch/4
  Constant/1 -> Multiport Switch/3
  Constant2/1 -> Multiport Switch/6
  Constant3/1 -> Multiport Switch/5
  Multiport Switch/1 -> Q/1
  Gain6/1 -> Sum2/1
  Constant6/1 -> Multiport Switch/9
  Gain8/1 -> Sum2/3
  Constant5/1 -> Multiport Switch/8
  Constant7/1 -> Multiport Switch/2
  Sum2/1 -> Multiport Switch/1
  Constant4/1 -> Multiport Switch/7
  Gain7/1 -> Sum2/2

== system DC_Loads_Lib/TRU DC Loads/Phasor/Calc PQ/Tuned/Filter ==
  In : Inport
  Gain : Gain  Gain=1/b
  Integrator : Integrator  InitialCondition=x_initial
  Sum : Sum  Inputs=|+-  InputSameDT=on  SaturateOnIntegerOverflow=on  OutDataTypeStr=Inherit: Same as first input
  Out : Outport  VectorParamsAs1DForOutWhenUnconnected=off
  wires:
  Gain/1 -> Out/1, Sum/2
  Integrator/1 -> Gain/1
  In/1 -> Sum/1
  Sum/1 -> Integrator/1
